simulink model "case9"  (R2024b)
settings: Solver=FixedStepAuto  StartTime=0  StopTime=1  FixedStep=1e-7  RelTol=1e-3
values from neighbouring files (symbols this model uses):
  SG_D_1_D = 0.01056    [IEEE9_case_parameters.m]    (also in case1_parameters.m; case2_parameters.m; case3_parameters.m; case4_parameters.m)
  SG_D_1_EnableSaturation = 0    [IEEE9_case_parameters.m]    (also in case1_parameters.m; case2_parameters.m; case3_parameters.m; case4_parameters.m)
  SG_D_1_f0 = 60    [IEEE9_case_parameters.m]    (also in case1_parameters.m; case2_parameters.m; case3_parameters.m; case4_parameters.m)
  SG_D_1_H = 7.5    [IEEE9_case_parameters.m]    (also in case1_parameters.m; case2_parameters.m; case3_parameters.m; case4_parameters.m)
  SG_D_1_K_A = 20    [IEEE9_case_parameters.m]    (also in case1_parameters.m; case2_parameters.m; case3_parameters.m; case4_parameters.m)
  SG_D_1_K_E = 1.000000e+1    (= 10)    [IEEE9_case_parameters.m]    (also in case1_parameters.m; case2_parameters.m; case3_parameters.m; case4_parameters.m)
  SG_D_1_K_F = 2.363    [IEEE9_case_parameters.m]    (also in case1_parameters.m; case2_parameters.m; case3_parameters.m; case4_parameters.m)
  SG_D_1_K_s = 0.5    [IEEE9_case_parameters.m]    (also in case1_parameters.m = 5; case2_parameters.m = 5; case3_parameters.m = 5; case4_parameters.m = 5)
  SG_D_1_R_a = 0.001088    [IEEE9_case_parameters.m]    (also in case1_parameters.m; case2_parameters.m; case3_parameters.m; case4_parameters.m)
  SG_D_1_S_A = 1    [IEEE9_case_parameters.m]    (also in case1_parameters.m; case2_parameters.m; case3_parameters.m; case4_parameters.m)
  SG_D_1_S_B = 0.103    [IEEE9_case_parameters.m]    (also in case1_parameters.m; case2_parameters.m; case3_parameters.m; case4_parameters.m)
  SG_D_1_S_N = 10.659857    [IEEE9_case_parameters.m]    (also in case1_parameters.m; case2_parameters.m; case3_parameters.m; case4_parameters.m)
  SG_D_1_SpeedPara = 200    [IEEE9_case_parameters.m]    (also in case1_parameters.m; case2_parameters.m; case3_parameters.m; case4_parameters.m)
  SG_D_1_T_0 = 0.720173    [IEEE9_case_parameters.m]    (also in case1_parameters.m = 0.755522; case2_parameters.m = 0.808931; case3_parameters.m = 0.869402; case4_parameters.m = 0.729316)
  SG_D_1_T_1 = 0.3    [IEEE9_case_parameters.m]    (also in case1_parameters.m; case2_parameters.m; case3_parameters.m; case4_parameters.m)
  SG_D_1_T_2 = 0.05    [IEEE9_case_parameters.m]    (also in case1_parameters.m; case2_parameters.m; case3_parameters.m; case4_parameters.m)
  SG_D_1_T_3 = 0.02    [IEEE9_case_parameters.m]    (also in case1_parameters.m; case2_parameters.m; case3_parameters.m; case4_parameters.m)
  SG_D_1_T_4 = 0.005    [IEEE9_case_parameters.m]    (also in case1_parameters.m; case2_parameters.m; case3_parameters.m; case4_parameters.m)
  SG_D_1_T_A = 0.02    [IEEE9_case_parameters.m]    (also in case1_parameters.m; case2_parameters.m; case3_parameters.m; case4_parameters.m)
  SG_D_1_T_dd = 8.000000e+0    (= 8)    [IEEE9_case_parameters.m]    (also in case1_parameters.m; case2_parameters.m; case3_parameters.m; case4_parameters.m)
  SG_D_1_T_ddd = 0.04    [IEEE9_case_parameters.m]    (also in case1_parameters.m; case2_parameters.m; case3_parameters.m; case4_parameters.m)
  SG_D_1_T_E = 0.314    [IEEE9_case_parameters.m]    (also in case1_parameters.m; case2_parameters.m; case3_parameters.m; case4_parameters.m)
  SG_D_1_T_F = 0.35    [IEEE9_case_parameters.m]    (also in case1_parameters.m; case2_parameters.m; case3_parameters.m; case4_parameters.m)
  SG_D_1_T_qd = 0.8    [IEEE9_case_parameters.m]    (also in case1_parameters.m; case2_parameters.m; case3_parameters.m; case4_parameters.m)
  SG_D_1_T_qdd = 0.02    [IEEE9_case_parameters.m]    (also in case1_parameters.m; case2_parameters.m; case3_parameters.m; case4_parameters.m)
  SG_D_1_T_speed = 0.1    [IEEE9_case_parameters.m]    (also in case1_parameters.m = 200; case2_parameters.m = 200; case3_parameters.m = 200; case4_parameters.m = 200)
  SG_D_1_T_w = 0.5    [IEEE9_case_parameters.m]    (also in case1_parameters.m; case2_parameters.m; case3_parameters.m; case4_parameters.m)
  SG_D_1_V_ref = 1.990276    [IEEE9_case_parameters.m]    (also in case1_parameters.m = 2.042296; case2_parameters.m = 2.051388; case3_parameters.m = 2.089584; case4_parameters.m = 2.01845)
  SG_D_1_w_ref = 376.991118    [IEEE9_case_parameters.m]    (also in case1_parameters.m; case2_parameters.m; case3_parameters.m; case4_parameters.m)
  SG_D_1_wb = 6.000000e+1    (= 60)    [IEEE9_case_parameters.m]    (also in case1_parameters.m; case2_parameters.m; case3_parameters.m; case4_parameters.m)
  SG_D_1_x_d = 1.9    [IEEE9_case_parameters.m]    (also in case1_parameters.m; case2_parameters.m; case3_parameters.m; case4_parameters.m)
  SG_D_1_x_dd = 0.302    [IEEE9_case_parameters.m]    (also in case1_parameters.m; case2_parameters.m; case3_parameters.m; case4_parameters.m)
  SG_D_1_x_ddd = 0.204    [IEEE9_case_parameters.m]    (also in case1_parameters.m; case2_parameters.m; case3_parameters.m; case4_parameters.m)
  SG_D_1_x_l = 0.05    [IEEE9_case_parameters.m]    (also in case1_parameters.m; case2_parameters.m; case3_parameters.m; case4_parameters.m)
  SG_D_1_x_q = 1.3    [IEEE9_case_parameters.m]    (also in case1_parameters.m; case2_parameters.m; case3_parameters.m; case4_parameters.m)
  SG_D_1_x_qd = 0.5    [IEEE9_case_parameters.m]    (also in case1_parameters.m; case2_parameters.m; case3_parameters.m; case4_parameters.m)
  SG_D_1_x_qdd = 0.3    [IEEE9_case_parameters.m]    (also in case1_parameters.m; case2_parameters.m; case3_parameters.m; case4_parameters.m)
  SG_D_2_D = 0.02    [IEEE9_case_parameters.m]    (also in case1_parameters.m; case2_parameters.m; case3_parameters.m; case4_parameters.m)
  SG_D_2_EnableSaturation = 0    [IEEE9_case_parameters.m]    (also in case1_parameters.m; case2_parameters.m; case3_parameters.m; case4_parameters.m)
  SG_D_2_f0 = 60    [IEEE9_case_parameters.m]    (also in case1_parameters.m; case2_parameters.m; case3_parameters.m; case4_parameters.m)
  SG_D_2_H = 8.000000e+0    (= 8)    [IEEE9_case_parameters.m]    (also in case1_parameters.m; case2_parameters.m; case3_parameters.m; case4_parameters.m)
  SG_D_2_K_A = 20    [IEEE9_case_parameters.m]    (also in case1_parameters.m; case2_parameters.m; case3_parameters.m; case4_parameters.m)
  SG_D_2_K_E = 1.000000e+1    (= 10)    [IEEE9_case_parameters.m]    (also in case1_parameters.m; case2_parameters.m; case3_parameters.m; case4_parameters.m)
  SG_D_2_K_F = 2.363    [IEEE9_case_parameters.m]    (also in case1_parameters.m; case2_parameters.m; case3_parameters.m; case4_parameters.m)
  SG_D_2_K_s = 0.5    [IEEE9_case_parameters.m]    (also in case1_parameters.m = 4; case2_parameters.m = 4; case3_parameters.m = 4; case4_parameters.m = 4)
  SG_D_2_R_a = 0.001088    [IEEE9_case_parameters.m]    (also in case1_parameters.m; case2_parameters.m; case3_parameters.m; case4_parameters.m)
  SG_D_2_S_A = 1    [IEEE9_case_parameters.m]    (also in case1_parameters.m; case2_parameters.m; case3_parameters.m; case4_parameters.m)
  SG_D_2_S_B = 0.103    [IEEE9_case_parameters.m]    (also in case1_parameters.m; case2_parameters.m; case3_parameters.m; case4_parameters.m)
  SG_D_2_S_N = 10.659857    [IEEE9_case_parameters.m]    (also in case1_parameters.m; case2_parameters.m; case3_parameters.m; case4_parameters.m)
  SG_D_2_SpeedPara = 200    [IEEE9_case_parameters.m]    (also in case1_parameters.m; case2_parameters.m; case3_parameters.m; case4_parameters.m)
  SG_D_2_T_0 = 1.632913    [IEEE9_case_parameters.m]    (also in case1_parameters.m = 1.632925; case2_parameters.m = 1.632915; case3_parameters.m = 1.632914; case4_parameters.m = 1.632927)
  SG_D_2_T_1 = 0.2    [IEEE9_case_parameters.m]    (also in case1_parameters.m; case2_parameters.m; case3_parameters.m; case4_parameters.m)
  SG_D_2_T_2 = 0.05    [IEEE9_case_parameters.m]    (also in case1_parameters.m; case2_parameters.m; case3_parameters.m; case4_parameters.m)
  SG_D_2_T_3 = 0.02    [IEEE9_case_parameters.m]    (also in case1_parameters.m; case2_parameters.m; case3_parameters.m; case4_parameters.m)
  SG_D_2_T_4 = 0.005    [IEEE9_case_parameters.m]    (also in case1_parameters.m; case2_parameters.m; case3_parameters.m; case4_parameters.m)
  SG_D_2_T_A = 0.02    [IEEE9_case_parameters.m]    (also in case1_parameters.m; case2_parameters.m; case3_parameters.m; case4_parameters.m)
  SG_D_2_T_dd = 7.9    [IEEE9_case_parameters.m]    (also in case1_parameters.m; case2_parameters.m; case3_parameters.m; case4_parameters.m)
  SG_D_2_T_ddd = 0.04    [IEEE9_case_parameters.m]    (also in case1_parameters.m; case2_parameters.m; case3_parameters.m; case4_parameters.m)
  SG_D_2_T_E = 0.314    [IEEE9_case_parameters.m]    (also in case1_parameters.m; case2_parameters.m; case3_parameters.m; case4_parameters.m)
  SG_D_2_T_F = 0.35    [IEEE9_case_parameters.m]    (also in case1_parameters.m; case2_parameters.m; case3_parameters.m; case4_parameters.m)
  SG_D_2_T_qd = 0.8    [IEEE9_case_parameters.m]    (also in case1_parameters.m; case2_parameters.m; case3_parameters.m; case4_parameters.m)
  SG_D_2_T_qdd = 0.015    [IEEE9_case_parameters.m]    (also in case1_parameters.m; case2_parameters.m; case3_parameters.m; case4_parameters.m)
  SG_D_2_T_speed = 0.1    [IEEE9_case_parameters.m]    (also in case1_parameters.m = 150; case2_parameters.m = 150; case3_parameters.m = 150; case4_parameters.m = 150)
  SG_D_2_T_w = 0.35    [IEEE9_case_parameters.m]    (also in case1_parameters.m; case2_parameters.m; case3_parameters.m; case4_parameters.m)
  SG_D_2_V_ref = 2.58547    [IEEE9_case_parameters.m]    (also in case1_parameters.m = 2.597896; case2_parameters.m = 2.587136; case3_parameters.m = 2.586042; case4_parameters.m = 2.599679)
  SG_D_2_w_ref = 376.991118    [IEEE9_case_parameters.m]    (also in case1_parameters.m; case2_parameters.m; case3_parameters.m; case4_parameters.m)
  SG_D_2_wb = 6.000000e+1    (= 60)    [IEEE9_case_parameters.m]    (also in case1_parameters.m; case2_parameters.m; case3_parameters.m; case4_parameters.m)
  SG_D_2_x_d = 1.8    [IEEE9_case_parameters.m]    (also in case1_parameters.m; case2_parameters.m; case3_parameters.m; case4_parameters.m)
  SG_D_2_x_dd = 0.302    [IEEE9_case_parameters.m]    (also in case1_parameters.m; case2_parameters.m; case3_parameters.m; case4_parameters.m)
  SG_D_2_x_ddd = 0.204    [IEEE9_case_parameters.m]    (also in case1_parameters.m; case2_parameters.m; case3_parameters.m; case4_parameters.m)
  SG_D_2_x_l = 0.05    [IEEE9_case_parameters.m]    (also in case1_parameters.m; case2_parameters.m; case3_parameters.m; case4_parameters.m)
  SG_D_2_x_q = 1.25    [IEEE9_case_parameters.m]    (also in case1_parameters.m; case2_parameters.m; case3_parameters.m; case4_parameters.m)
  SG_D_2_x_qd = 0.5    [IEEE9_case_parameters.m]    (also in case1_parameters.m; case2_parameters.m; case3_parameters.m; case4_parameters.m)
  SG_D_2_x_qdd = 0.3    [IEEE9_case_parameters.m]    (also in case1_parameters.m; case2_parameters.m; case3_parameters.m; case4_parameters.m)
  SG_D_3_D = 0.02    [IEEE9_case_parameters.m]    (also in case1_parameters.m; case2_parameters.m; case3_parameters.m; case4_parameters.m)
  SG_D_3_EnableSaturation = 0    [IEEE9_case_parameters.m]    (also in case1_parameters.m; case2_parameters.m; case3_parameters.m; case4_parameters.m)
  SG_D_3_f0 = 60    [IEEE9_case_parameters.m]    (also in case1_parameters.m; case2_parameters.m; case3_parameters.m; case4_parameters.m)
  SG_D_3_H = 7.7    [IEEE9_case_parameters.m]    (also in case1_parameters.m; case2_parameters.m; case3_parameters.m; case4_parameters.m)
  SG_D_3_K_A = 20    [IEEE9_case_parameters.m]    (also in case1_parameters.m; case2_parameters.m; case3_parameters.m; case4_parameters.m)
  SG_D_3_K_E = 1.000000e+1    (= 10)    [IEEE9_case_parameters.m]    (also in case1_parameters.m; case2_parameters.m; case3_parameters.m; case4_parameters.m)
  SG_D_3_K_F = 2.363    [IEEE9_case_parameters.m]    (also in case1_parameters.m; case2_parameters.m; case3_parameters.m; case4_parameters.m)
  SG_D_3_K_s = 0.2    [IEEE9_case_parameters.m]    (also in case1_parameters.m = 2; case2_parameters.m = 2; case3_parameters.m = 2; case4_parameters.m = 2)
  SG_D_3_R_a = 0.001088    [IEEE9_case_parameters.m]    (also in case1_parameters.m; case2_parameters.m; case3_parameters.m; case4_parameters.m)
  SG_D_3_S_A = 1    [IEEE9_case_parameters.m]    (also in case1_parameters.m; case2_parameters.m; case3_parameters.m; case4_parameters.m)
  SG_D_3_S_B = 0.103    [IEEE9_case_parameters.m]    (also in case1_parameters.m; case2_parameters.m; case3_parameters.m; case4_parameters.m)
  SG_D_3_S_N = 10.659857    [IEEE9_case_parameters.m]    (also in case1_parameters.m; case2_parameters.m; case3_parameters.m; case4_parameters.m)
  SG_D_3_SpeedPara = 200    [IEEE9_case_parameters.m]    (also in case1_parameters.m; case2_parameters.m; case3_parameters.m; case4_parameters.m)
  SG_D_3_T_0 = 0.850788    [IEEE9_case_parameters.m]    (also in case1_parameters.m = 0.850786; case2_parameters.m = 0.850787; case3_parameters.m; case4_parameters.m = 0.850786)
  SG_D_3_T_1 = 0.2    [IEEE9_case_parameters.m]    (also in case1_parameters.m; case2_parameters.m; case3_parameters.m; case4_parameters.m)
  SG_D_3_T_2 = 0.05    [IEEE9_case_parameters.m]    (also in case1_parameters.m; case2_parameters.m; case3_parameters.m; case4_parameters.m)
  SG_D_3_T_3 = 0.02    [IEEE9_case_parameters.m]    (also in case1_parameters.m; case2_parameters.m; case3_parameters.m; case4_parameters.m)
  SG_D_3_T_4 = 0.005    [IEEE9_case_parameters.m]    (also in case1_parameters.m; case2_parameters.m; case3_parameters.m; case4_parameters.m)
  SG_D_3_T_A = 0.02    [IEEE9_case_parameters.m]    (also in case1_parameters.m; case2_parameters.m; case3_parameters.m; case4_parameters.m)
  SG_D_3_T_dd = 8.1    [IEEE9_case_parameters.m]    (also in case1_parameters.m; case2_parameters.m; case3_parameters.m; case4_parameters.m)
  SG_D_3_T_ddd = 0.04    [IEEE9_case_parameters.m]    (also in case1_parameters.m; case2_parameters.m; case3_parameters.m; case4_parameters.m)
  SG_D_3_T_E = 0.314    [IEEE9_case_parameters.m]    (also in case1_parameters.m; case2_parameters.m; case3_parameters.m; case4_parameters.m)
  SG_D_3_T_F = 0.35    [IEEE9_case_parameters.m]    (also in case1_parameters.m; case2_parameters.m; case3_parameters.m; case4_parameters.m)
  SG_D_3_T_qd = 0.8    [IEEE9_case_parameters.m]    (also in case1_parameters.m; case2_parameters.m; case3_parameters.m; case4_parameters.m)
  SG_D_3_T_qdd = 0.015    [IEEE9_case_parameters.m]    (also in case1_parameters.m; case2_parameters.m; case3_parameters.m; case4_parameters.m)
  SG_D_3_T_speed = 0.1    [IEEE9_case_parameters.m]    (also in case1_parameters.m = 180; case2_parameters.m = 180; case3_parameters.m = 180; case4_parameters.m = 180)
  SG_D_3_T_w = 0.4    [IEEE9_case_parameters.m]    (also in case1_parameters.m; case2_parameters.m; case3_parameters.m; case4_parameters.m)
  SG_D_3_V_ref = 1.892727    [IEEE9_case_parameters.m]    (also in case1_parameters.m = 1.906439; case2_parameters.m = 1.895535; case3_parameters.m = 1.892105; case4_parameters.m = 1.906598)
  SG_D_3_w_ref = 376.991118    [IEEE9_case_parameters.m]    (also in case1_parameters.m; case2_parameters.m; case3_parameters.m; case4_parameters.m)
  SG_D_3_wb = 6.000000e+1    (= 60)    [IEEE9_case_parameters.m]    (also in case1_parameters.m; case2_parameters.m; case3_parameters.m; case4_parameters.m)
  SG_D_3_x_d = 1.85    [IEEE9_case_parameters.m]    (also in case1_parameters.m; case2_parameters.m; case3_parameters.m; case4_parameters.m)
  SG_D_3_x_dd = 0.302    [IEEE9_case_parameters.m]    (also in case1_parameters.m; case2_parameters.m; case3_parameters.m; case4_parameters.m)
  SG_D_3_x_ddd = 0.204    [IEEE9_case_parameters.m]    (also in case1_parameters.m; case2_parameters.m; case3_parameters.m; case4_parameters.m)
  SG_D_3_x_l = 0.05    [IEEE9_case_parameters.m]    (also in case1_parameters.m; case2_parameters.m; case3_parameters.m; case4_parameters.m)
  SG_D_3_x_q = 1.2    [IEEE9_case_parameters.m]    (also in case1_parameters.m; case2_parameters.m; case3_parameters.m; case4_parameters.m)
  SG_D_3_x_qd = 0.5    [IEEE9_case_parameters.m]    (also in case1_parameters.m; case2_parameters.m; case3_parameters.m; case4_parameters.m)
  SG_D_3_x_qdd = 0.3    [IEEE9_case_parameters.m]    (also in case1_parameters.m; case2_parameters.m; case3_parameters.m; case4_parameters.m)
(part 6 of 12)

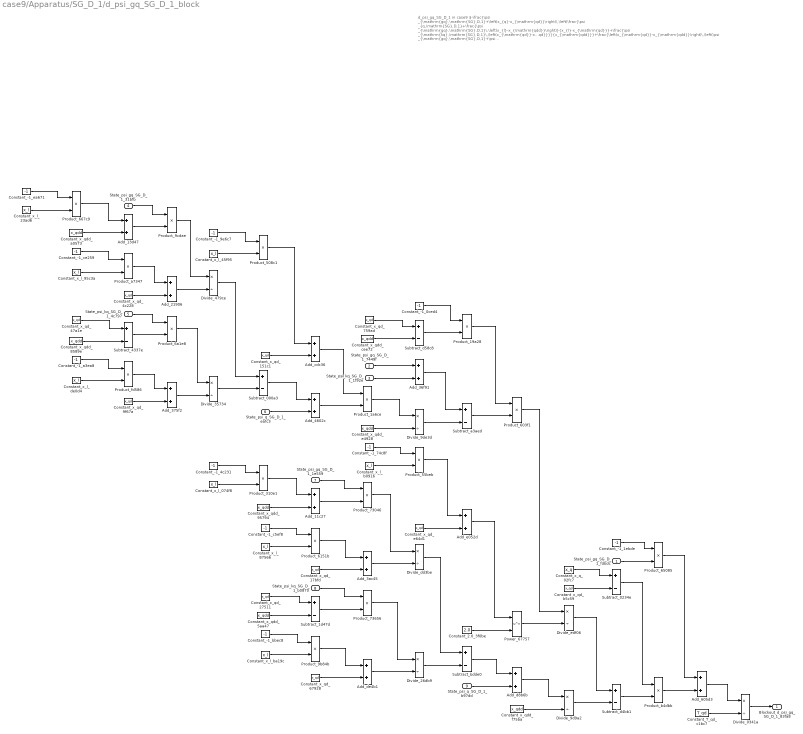
== system case9/Apparatus/SG_D_1/d_psi_gq_SG_D_1_block ==
  note: d_psi_gq_SG_D_1 in case9
      | $-\frac{\psi _{\mathrm{gq},\mathrm{SG},D,1}+\left(x_{q}-x_{\mathrm{qd}}\right)\,\left(\frac{\psi _{q,\mathrm{SG},D,1}+\frac{\psi _{\mathrm{gq},\mathrm{SG},D,1}\,\left(x_{l}-x_{\mathrm{qdd}}\right)}{x_{l}-x_{\mathrm{qd}}}+\frac{\psi _{\mathrm{kq},\mathrm{SG},D,1}\,\left(x_{\mathrm{qd}}-x_{\mathrm{qdd}}\right)}{x_{l}-x_{\mathrm{qd}}}}{x_{\mathrm{qdd}}}+\frac{\left(x_{\mathrm{qd}}-x_{\mathrm{qdd}}\right)\,\left(\psi _{\mathrm{gq},\mathrm{SG},D,1}+\psi _{\mathrm{kq},\mathrm{SG},D,1}+\frac{\left(x_{l}-x_{\mathrm{qd}}\right)\,\left(\psi _{q,\mathrm{SG},D,1}+\frac{\psi _{\mathrm{gq},\mathrm{SG},D,1}\,\left(x_{l}-x_{\mathrm{qdd}}\right)}{x_{l}-x_{\mathrm{qd}}}+\frac{\psi _{\mathrm{kq},\mathrm{SG},D,1}\,\left(x_{\mathrm{qd}}-x_{\mathrm{qdd}}\right)}{x_{l}-x_{\mathrm{qd}}}\right)}{x_{\mathrm{qdd}}}\right)}{{\left(x_{l}-x_{\mathrm{qd}}\right)}^2}\right)}{T_{\mathrm{qd}}}$
      | Automatically generated on 2025-10-31 19:34:40 .
  State_psi_gq_SG_D_1_fdbdc : Inport
  State_psi_gq_SG_D_1_7449f : Inport  Port=2
  State_psi_kq_SG_D_1_1f92e : Inport  Port=3
  State_psi_gq_SG_D_1_31bfb : Inport  Port=4
  State_psi_kq_SG_D_1_4c797 : Inport  Port=5
  State_psi_q_SG_D_1_eafc3 : Inport  Port=6
  State_psi_gq_SG_D_1_1e559 : Inport  Port=7
  State_psi_kq_SG_D_1_b0870 : Inport  Port=8
  State_psi_q_SG_D_1_b97dd : Inport  Port=9
  Add_11c27 : Sum
  Add_13d47 : Sum
  Add_21906 : Sum
  Add_36f91 : Sum
  Add_375f2 : Sum
  Add_3ac45 : Sum
  Add_4602c : Sum
  Add_605d3 : Sum
  Add_cdc36 : Sum
  Add_d8b6b : Sum
  Add_de4b1 : Sum
  Add_e052d : Sum
  Constant_-1_0ced4 : Constant  Value=-1
  Constant_-1_1ebde : Constant  Value=-1
  Constant_-1_4c231 : Constant  Value=-1
  Constant_-1_74c8f : Constant  Value=-1
  Constant_-1_9e6c7 : Constant  Value=-1
  Constant_-1_a3ea8 : Constant  Value=-1
  Constant_-1_bbec8 : Constant  Value=-1
  Constant_-1_c5ef8 : Constant  Value=-1
  Constant_-1_ce259 : Constant  Value=-1
  Constant_-1_ea671 : Constant  Value=-1
  Constant_2.0_3f0be : Constant  Value=2.0
  Constant_T_qd_c1bc7 : Constant  Value=T_qd
  Constant_x_l_074f8 : Constant  Value=x_l
  Constant_x_l_23ad6 : Constant  Value=x_l
  Constant_x_l_45f95 : Constant  Value=x_l
  Constant_x_l_87566 : Constant  Value=x_l
  Constant_x_l_95c3a : Constant  Value=x_l
  Constant_x_l_b0916 : Constant  Value=x_l
  Constant_x_l_ba19c : Constant  Value=x_l
  Constant_x_l_de0d4 : Constant  Value=x_l
  Constant_x_q_02fc7 : Constant  Value=x_q
  Constant_x_qd_151c1 : Constant  Value=x_qd
  Constant_x_qd_17bfd : Constant  Value=x_qd
  Constant_x_qd_27511 : Constant  Value=x_qd
  Constant_x_qd_47a1e : Constant  Value=x_qd
  Constant_x_qd_4c228 : Constant  Value=x_qd
  Constant_x_qd_67928 : Constant  Value=x_qd
  Constant_x_qd_759ad : Constant  Value=x_qd
  Constant_x_qd_9f67a : Constant  Value=x_qd
  Constant_x_qd_b5c59 : Constant  Value=x_qd
  Constant_x_qd_e64d1 : Constant  Value=x_qd
  Constant_x_qdd_5aa47 : Constant  Value=x_qdd
  Constant_x_qdd_8589e : Constant  Value=x_qdd
  Constant_x_qdd_95794 : Constant  Value=x_qdd
  Constant_x_qdd_a0573 : Constant  Value=x_qdd
  Constant_x_qdd_cee72 : Constant  Value=x_qdd
  Constant_x_qdd_e4928 : Constant  Value=x_qdd
  Constant_x_qdd_f75ba : Constant  Value=x_qdd
  Divide_0341a : Product  Inputs=*/
  Divide_26db9 : Product  Inputs=*/
  Divide_35734 : Product  Inputs=*/
  Divide_479ce : Product  Inputs=*/
  Divide_9d9a2 : Product  Inputs=*/
  Divide_9de3d : Product  Inputs=*/
  Divide_dd3be : Product  Inputs=*/
  Divide_edf06 : Product  Inputs=*/
  Power_67757 : Math  Operator=pow
  Product_19a28 : Product
  Product_1a6ce : Product
  Product_310e1 : Product
  Product_508c1 : Product
  Product_55beb : Product
  Product_603f1 : Product
  Product_6151b : Product
  Product_65085 : Product
  Product_667c9 : Product
  Product_6a1e8 : Product
  Product_73046 : Product
  Product_73656 : Product
  Product_9b84b : Product
  Product_9cdae : Product
  Product_a7347 : Product
  Product_b4dbb : Product
  Product_fd586 : Product
  Subtract_000a3 : Sum  Inputs=+-
  Subtract_0234e : Sum  Inputs=+-
  Subtract_1d47d : Sum  Inputs=+-
  Subtract_4337e : Sum  Inputs=+-
  Subtract_a3aed : Sum  Inputs=+-
  Subtract_bdde0 : Sum  Inputs=+-
  Subtract_d4bb1 : Sum  Inputs=+-
  Subtract_d58c8 : Sum  Inputs=+-
  Blockout_d_psi_gq_SG_D_1_83fa8 : Outport
  wires:
  State_psi_gq_SG_D_1_31bfb/1 -> Product_9cdae/1
  Constant_-1_ce259/1 -> Product_a7347/1
  Divide_479ce/1 -> Subtract_000a3/1
  Add_21906/1 -> Divide_479ce/2
  Product_667c9/1 -> Add_13d47/1
  Constant_x_qd_151c1/1 -> Add_cdc36/2
  Constant_-1_ea671/1 -> Product_667c9/1
  Constant_x_qdd_a0573/1 -> Add_13d47/2
  Constant_x_l_95c3a/1 -> Product_a7347/2
  Constant_x_l_23ad6/1 -> Product_667c9/2
  Constant_-1_a3ea8/1 -> Product_fd586/1
  Constant_x_qd_47a1e/1 -> Subtract_4337e/1
  Constant_x_qdd_e4928/1 -> Divide_9de3d/2
  Constant_x_l_de0d4/1 -> Product_fd586/2
  Constant_x_qdd_8589e/1 -> Subtract_4337e/2
  Subtract_000a3/1 -> Add_4602c/1
  Add_13d47/1 -> Product_9cdae/2
  Product_9cdae/1 -> Divide_479ce/1
  Product_a7347/1 -> Add_21906/1
  Constant_x_qd_4c228/1 -> Add_21906/2
  State_psi_kq_SG_D_1_4c797/1 -> Product_6a1e8/1
  Product_fd586/1 -> Add_375f2/1
  Subtract_4337e/1 -> Product_6a1e8/2
  Constant_x_qd_9f67a/1 -> Add_375f2/2
  Product_6a1e8/1 -> Divide_35734/1
  Add_375f2/1 -> Divide_35734/2
  Constant_-1_0ced4/1 -> Product_19a28/1
  Constant_-1_9e6c7/1 -> Product_508c1/1
  Add_3ac45/1 -> Divide_dd3be/2
  Product_9b84b/1 -> Add_de4b1/1
  Subtract_1d47d/1 -> Product_73656/2
  Constant_x_l_45f95/1 -> Product_508c1/2
  Divide_35734/1 -> Subtract_000a3/2
  Subtract_0234e/1 -> Product_b4dbb/1
  Constant_-1_74c8f/1 -> Product_55beb/1
  Constant_-1_4c231/1 -> Product_310e1/1
  Constant_x_l_b0916/1 -> Product_55beb/2
  Constant_x_l_074f8/1 -> Product_310e1/2
  Constant_x_qd_17bfd/1 -> Add_3ac45/2
  Product_508c1/1 -> Add_cdc36/1
  State_psi_q_SG_D_1_eafc3/1 -> Add_4602c/2
  Product_310e1/1 -> Add_11c27/1
  Constant_x_qdd_95794/1 -> Add_11c27/2
  Constant_-1_c5ef8/1 -> Product_6151b/1
  Constant_x_qd_67928/1 -> Add_de4b1/2
  Add_cdc36/1 -> Product_1a6ce/1
  Constant_x_l_87566/1 -> Product_6151b/2
  Constant_-1_bbec8/1 -> Product_9b84b/1
  Constant_x_qd_27511/1 -> Subtract_1d47d/1
  Product_1a6ce/1 -> Divide_9de3d/1
  Constant_x_l_ba19c/1 -> Product_9b84b/2
  Divide_edf06/1 -> Subtract_d4bb1/1
  Constant_x_qdd_5aa47/1 -> Subtract_1d47d/2
  Add_4602c/1 -> Product_1a6ce/2
  State_psi_gq_SG_D_1_1e559/1 -> Product_73046/1
  Add_11c27/1 -> Product_73046/2
  Product_6151b/1 -> Add_3ac45/1
  State_psi_kq_SG_D_1_b0870/1 -> Product_73656/1
  Add_de4b1/1 -> Divide_26db9/2
  State_psi_gq_SG_D_1_7449f/1 -> Add_36f91/1
  Constant_x_qd_759ad/1 -> Subtract_d58c8/1
  Constant_x_qdd_cee72/1 -> Subtract_d58c8/2
  Product_73656/1 -> Divide_26db9/1
  State_psi_kq_SG_D_1_1f92e/1 -> Add_36f91/2
  Product_73046/1 -> Divide_dd3be/1
  Subtract_d58c8/1 -> Product_19a28/2
  Add_36f91/1 -> Subtract_a3aed/1
  Divide_9de3d/1 -> Subtract_a3aed/2
  Product_55beb/1 -> Add_e052d/1
  Constant_x_qd_e64d1/1 -> Add_e052d/2
  Divide_dd3be/1 -> Subtract_bdde0/1
  Divide_26db9/1 -> Subtract_bdde0/2
  Product_19a28/1 -> Product_603f1/1
  Subtract_a3aed/1 -> Product_603f1/2
  Add_e052d/1 -> Power_67757/1
  Constant_2.0_3f0be/1 -> Power_67757/2
  Subtract_bdde0/1 -> Add_d8b6b/1
  State_psi_q_SG_D_1_b97dd/1 -> Add_d8b6b/2
  Product_603f1/1 -> Divide_edf06/1
  Power_67757/1 -> Divide_edf06/2
  Add_d8b6b/1 -> Divide_9d9a2/1
  Constant_x_qdd_f75ba/1 -> Divide_9d9a2/2
  Constant_x_q_02fc7/1 -> Subtract_0234e/1
  Constant_x_qd_b5c59/1 -> Subtract_0234e/2
  Divide_9d9a2/1 -> Subtract_d4bb1/2
  Constant_-1_1ebde/1 -> Product_65085/1
  State_psi_gq_SG_D_1_fdbdc/1 -> Product_65085/2
  Subtract_d4bb1/1 -> Product_b4dbb/2
  Product_65085/1 -> Add_605d3/1
  Product_b4dbb/1 -> Add_605d3/2
  Add_605d3/1 -> Divide_0341a/1
  Constant_T_qd_c1bc7/1 -> Divide_0341a/2
  Divide_0341a/1 -> Blockout_d_psi_gq_SG_D_1_83fa8/1

== system case9/Apparatus/SG_D_1/d_psi_kq_SG_D_1_block ==
  note: d_psi_kq_SG_D_1 in case9
      | $-\frac{\psi _{\mathrm{gq},\mathrm{SG},D,1}+\psi _{\mathrm{kq},\mathrm{SG},D,1}+\frac{\left(x_{l}-x_{\mathrm{qd}}\right)\,\left(\psi _{q,\mathrm{SG},D,1}+\frac{\psi _{\mathrm{gq},\mathrm{SG},D,1}\,\left(x_{l}-x_{\mathrm{qdd}}\right)}{x_{l}-x_{\mathrm{qd}}}+\frac{\psi _{\mathrm{kq},\mathrm{SG},D,1}\,\left(x_{\mathrm{qd}}-x_{\mathrm{qdd}}\right)}{x_{l}-x_{\mathrm{qd}}}\right)}{x_{\mathrm{qdd}}}}{T_{\mathrm{qdd}}}$
      | Automatically generated on 2025-10-31 19:34:41 .
  State_psi_gq_SG_D_1_20359 : Inport
  State_psi_kq_SG_D_1_02235 : Inport  Port=2
  State_psi_gq_SG_D_1_5b14b : Inport  Port=3
  State_psi_kq_SG_D_1_1396d : Inport  Port=4
  State_psi_q_SG_D_1_e7314 : Inport  Port=5
  Add_06458 : Sum
  Add_873c5 : Sum
  Add_945ca : Sum
  Add_95636 : Sum
  Add_a65ed : Sum
  Add_bc1c6 : Sum
  Constant_-1_4b348 : Constant  Value=-1
  Constant_-1_66d13 : Constant  Value=-1
  Constant_-1_7eae6 : Constant  Value=-1
  Constant_-1_b006a : Constant  Value=-1
  Constant_-1_fe53d : Constant  Value=-1
  Constant_T_qdd_5e4e9 : Constant  Value=T_qdd
  Constant_x_l_2eef6 : Constant  Value=x_l
  Constant_x_l_461f2 : Constant  Value=x_l
  Constant_x_l_559ed : Constant  Value=x_l
  Constant_x_l_a9a58 : Constant  Value=x_l
  Constant_x_qd_1a100 : Constant  Value=x_qd
  Constant_x_qd_67afc : Constant  Value=x_qd
  Constant_x_qd_edeff : Constant  Value=x_qd
  Constant_x_qd_fdf31 : Constant  Value=x_qd
  Constant_x_qdd_400b6 : Constant  Value=x_qdd
  Constant_x_qdd_692c4 : Constant  Value=x_qdd
  Constant_x_qdd_be4c0 : Constant  Value=x_qdd
  Divide_2b43f : Product  Inputs=*/
  Divide_71da8 : Product  Inputs=*/
  Divide_bf59b : Product  Inputs=*/
  Divide_f6de6 : Product  Inputs=*/
  Product_0ba77 : Product
  Product_17ebc : Product
  Product_25d03 : Product
  Product_4de9c : Product
  Product_5fbf3 : Product
  Product_913de : Product
  Product_c66f6 : Product
  Product_d3303 : Product
  Subtract_28a94 : Sum  Inputs=+-
  Subtract_7a2c0 : Sum  Inputs=+-
  Subtract_9b8fd : Sum  Inputs=+-
  Blockout_d_psi_kq_SG_D_1_1846f : Outport
  wires:
  Product_25d03/1 -> Add_95636/1
  Constant_-1_66d13/1 -> Product_25d03/1
  Constant_x_l_2eef6/1 -> Product_25d03/2
  Constant_x_qdd_400b6/1 -> Add_95636/2
  Constant_-1_4b348/1 -> Product_d3303/1
  Constant_x_qd_1a100/1 -> Subtract_28a94/1
  Constant_x_qd_fdf31/1 -> Add_945ca/2
  Constant_-1_b006a/1 -> Product_17ebc/1
  Constant_x_l_461f2/1 -> Product_d3303/2
  Constant_x_qdd_be4c0/1 -> Subtract_28a94/2
  Constant_x_qd_67afc/1 -> Add_bc1c6/2
  Constant_x_l_a9a58/1 -> Product_17ebc/2
  Subtract_9b8fd/1 -> Add_06458/1
  Product_5fbf3/1 -> Subtract_9b8fd/1
  State_psi_gq_SG_D_1_5b14b/1 -> Product_c66f6/1
  Add_95636/1 -> Product_c66f6/2
  Product_17ebc/1 -> Add_a65ed/1
  Constant_x_qd_edeff/1 -> Add_a65ed/2
  State_psi_kq_SG_D_1_1396d/1 -> Product_0ba77/1
  Product_d3303/1 -> Add_bc1c6/1
  Subtract_28a94/1 -> Product_0ba77/2
  Product_c66f6/1 -> Divide_f6de6/1
  Add_a65ed/1 -> Divide_f6de6/2
  Product_0ba77/1 -> Divide_71da8/1
  Add_bc1c6/1 -> Divide_71da8/2
  Constant_-1_7eae6/1 -> Product_4de9c/1
  Constant_x_l_559ed/1 -> Product_4de9c/2
  Divide_f6de6/1 -> Subtract_7a2c0/1
  Divide_71da8/1 -> Subtract_7a2c0/2
  Product_4de9c/1 -> Add_945ca/1
  Add_873c5/1 -> Product_913de/2
  Subtract_7a2c0/1 -> Add_873c5/1
  State_psi_q_SG_D_1_e7314/1 -> Add_873c5/2
  Constant_-1_fe53d/1 -> Product_5fbf3/1
  State_psi_gq_SG_D_1_20359/1 -> Product_5fbf3/2
  Divide_2b43f/1 -> Add_06458/2
  Product_913de/1 -> Divide_2b43f/1
  Add_945ca/1 -> Product_913de/1
  State_psi_kq_SG_D_1_02235/1 -> Subtract_9b8fd/2
  Constant_x_qdd_692c4/1 -> Divide_2b43f/2
  Add_06458/1 -> Divide_bf59b/1
  Constant_T_qdd_5e4e9/1 -> Divide_bf59b/2
  Divide_bf59b/1 -> Blockout_d_psi_kq_SG_D_1_1846f/1

== system case9/Apparatus/SG_D_1/d_psi_q_SG_D_1_block ==
  note: d_psi_q_SG_D_1 in case9
      | $2\,\pi \,f_{0}\,\left(v_{d,\mathrm{SG},D,1}\,\cos\left(\theta _{\mathrm{SG},D,1}\right)+v_{q,\mathrm{SG},D,1}\,\sin\left(\theta _{\mathrm{SG},D,1}\right)-\frac{R_{a}\,\left(\psi _{q,\mathrm{SG},D,1}+\frac{\psi _{\mathrm{gq},\mathrm{SG},D,1}\,\left(x_{l}-x_{\mathrm{qdd}}\right)}{x_{l}-x_{\mathrm{qd}}}+\frac{\psi _{\mathrm{kq},\mathrm{SG},D,1}\,\left(x_{\mathrm{qd}}-x_{\mathrm{qdd}}\right)}{x_{l}-x_{\mathrm{qd}}}\right)}{x_{\mathrm{qdd}}}-\frac{\psi _{d,\mathrm{SG},D,1}\,w_{\mathrm{SG},D,1}}{2\,f_{0}\,\pi }\right)$
      | Automatically generated on 2025-10-31 19:34:37 .
  State_psi_gq_SG_D_1_e06cf : Inport
  State_psi_kq_SG_D_1_d4ed3 : Inport  Port=2
  State_psi_q_SG_D_1_8f107 : Inport  Port=3
  Input_v_d_SG_D_1_e85f7 : Inport  Port=4
  State_theta_SG_D_1_b63a1 : Inport  Port=5
  Input_v_q_SG_D_1_46a58 : Inport  Port=6
  State_theta_SG_D_1_fcbfe : Inport  Port=7
  State_psi_d_SG_D_1_9ece2 : Inport  Port=8
  State_w_SG_D_1_a0845 : Inport  Port=9
  Add_323c6 : Sum
  Add_583ae : Sum
  Add_6779d : Sum
  Add_6acf7 : Sum
  Add_b46b4 : Sum
  Constant_-1_024fb : Constant  Value=-1
  Constant_-1_6bd05 : Constant  Value=-1
  Constant_-1_9f485 : Constant  Value=-1
  Constant_-2.0_28195 : Constant  Value=-2.0
  Constant_2.0_387e6 : Constant  Value=2.0
  Constant_R_a_e430c : Constant  Value=R_a
  Constant_f0_73c2d : Constant  Value=f0
  Constant_f0_e8bd1 : Constant  Value=f0
  Constant_pi_9a496 : Constant  Value=pi
  Constant_pi_a35a0 : Constant  Value=pi
  Constant_x_l_7e967 : Constant  Value=x_l
  Constant_x_l_c6c0d : Constant  Value=x_l
  Constant_x_l_efad4 : Constant  Value=x_l
  Constant_x_qd_155b8 : Constant  Value=x_qd
  Constant_x_qd_2e84c : Constant  Value=x_qd
  Constant_x_qd_f4c16 : Constant  Value=x_qd
  Constant_x_qdd_91f68 : Constant  Value=x_qdd
  Constant_x_qdd_b22e8 : Constant  Value=x_qdd
  Constant_x_qdd_d86ff : Constant  Value=x_qdd
  Divide_09ba4 : Product  Inputs=*/
  Divide_15066 : Product  Inputs=*/
  Divide_3baef : Product  Inputs=*/
  Divide_3e22e : Product  Inputs=*/
  MathFunc_cos_5ad6c : Trigonometry  Operator=cos
  MathFunc_sin_42c9e : Trigonometry
  Product_2401e : Product
  Product_29cb7 : Product
  Product_2ec6b : Product
  Product_31a30 : Product
  Product_46fe9 : Product
  Product_4fd8e : Product
  Product_50d90 : Product
  Product_5e278 : Product
  Product_76f09 : Product
  Product_87948 : Product
  Product_8bfc0 : Product
  Product_97d6d : Product
  Product_c3375 : Product
  Product_f5b25 : Product
  Subtract_2f3d6 : Sum  Inputs=+-
  Subtract_e6a18 : Sum  Inputs=+-
  Subtract_ea955 : Sum  Inputs=+-
  Subtract_f36d7 : Sum  Inputs=+-
  Blockout_d_psi_q_SG_D_1_00fdb : Outport
  wires:
  Divide_3baef/1 -> Subtract_f36d7/1
  Product_76f09/1 -> Add_583ae/1
  Constant_x_l_c6c0d/1 -> Product_76f09/2
  Constant_-1_024fb/1 -> Product_76f09/1
  Constant_x_qdd_b22e8/1 -> Add_583ae/2
  Constant_x_l_7e967/1 -> Product_f5b25/2
  Constant_-1_9f485/1 -> Product_f5b25/1
  Constant_x_l_efad4/1 -> Product_97d6d/2
  Constant_x_qdd_91f68/1 -> Subtract_ea955/2
  State_psi_kq_SG_D_1_d4ed3/1 -> Product_8bfc0/1
  Constant_-1_6bd05/1 -> Product_97d6d/1
  Constant_x_qd_f4c16/1 -> Subtract_ea955/1
  State_psi_gq_SG_D_1_e06cf/1 -> Product_5e278/1
  Product_31a30/1 -> Blockout_d_psi_q_SG_D_1_00fdb/1
  Subtract_f36d7/1 -> Add_6acf7/1
  Product_5e278/1 -> Divide_3baef/1
  Add_583ae/1 -> Product_5e278/2
  Divide_3e22e/1 -> Subtract_f36d7/2
  Product_f5b25/1 -> Add_6779d/1
  Constant_x_qd_155b8/1 -> Add_6779d/2
  Constant_-2.0_28195/1 -> Product_c3375/1
  Product_8bfc0/1 -> Divide_3e22e/1
  Product_97d6d/1 -> Add_323c6/1
  Subtract_ea955/1 -> Product_8bfc0/2
  Constant_x_qd_2e84c/1 -> Add_323c6/2
  Add_6779d/1 -> Divide_3baef/2
  Add_323c6/1 -> Divide_3e22e/2
  Constant_f0_73c2d/1 -> Product_29cb7/2
  State_psi_q_SG_D_1_8f107/1 -> Add_6acf7/2
  Product_46fe9/1 -> Product_4fd8e/1
  Constant_R_a_e430c/1 -> Product_87948/1
  Product_4fd8e/1 -> Divide_09ba4/2
  Product_87948/1 -> Divide_15066/1
  Add_6acf7/1 -> Product_87948/2
  State_theta_SG_D_1_b63a1/1 -> MathFunc_cos_5ad6c/1
  Input_v_d_SG_D_1_e85f7/1 -> Product_2ec6b/1
  Constant_x_qdd_d86ff/1 -> Divide_15066/2
  MathFunc_cos_5ad6c/1 -> Product_2ec6b/2
  State_theta_SG_D_1_fcbfe/1 -> MathFunc_sin_42c9e/1
  Divide_15066/1 -> Subtract_2f3d6/1
  Constant_2.0_387e6/1 -> Product_46fe9/1
  State_w_SG_D_1_a0845/1 -> Product_2401e/2
  Constant_pi_9a496/1 -> Product_46fe9/2
  Subtract_e6a18/1 -> Add_b46b4/1
  Product_2ec6b/1 -> Subtract_2f3d6/2
  Divide_09ba4/1 -> Add_b46b4/2
  Input_v_q_SG_D_1_46a58/1 -> Product_50d90/1
  MathFunc_sin_42c9e/1 -> Product_50d90/2
  Product_50d90/1 -> Subtract_e6a18/2
  State_psi_d_SG_D_1_9ece2/1 -> Product_2401e/1
  Constant_f0_e8bd1/1 -> Product_4fd8e/2
  Constant_pi_a35a0/1 -> Product_c3375/2
  Subtract_2f3d6/1 -> Subtract_e6a18/1
  Product_2401e/1 -> Divide_09ba4/1
  Product_c3375/1 -> Product_29cb7/1
  Product_29cb7/1 -> Product_31a30/1
  Add_b46b4/1 -> Product_31a30/2

== system case9/Apparatus/SG_D_1/d_theta_SG_D_1_block ==
  note: d_theta_SG_D_1 in case9
      | $w_{\mathrm{SG},D,1}-2\,\pi \,f_{0}$
      | Automatically generated on 2025-10-31 19:34:43 .
  State_w_SG_D_1_c5d1e : Inport
  Add_b1f62 : Sum
  Constant_-2.0_b7139 : Constant  Value=-2.0
  Constant_f0_a2466 : Constant  Value=f0
  Constant_pi_6dd0a : Constant  Value=pi
  Product_2a34f : Product
  Product_c6ee4 : Product
  Blockout_d_theta_SG_D_1_9a995 : Outport
  wires:
  State_w_SG_D_1_c5d1e/1 -> Add_b1f62/2
  Constant_-2.0_b7139/1 -> Product_c6ee4/1
  Constant_f0_a2466/1 -> Product_2a34f/2
  Constant_pi_6dd0a/1 -> Product_c6ee4/2
  Product_2a34f/1 -> Add_b1f62/1
  Product_c6ee4/1 -> Product_2a34f/1
  Add_b1f62/1 -> Blockout_d_theta_SG_D_1_9a995/1

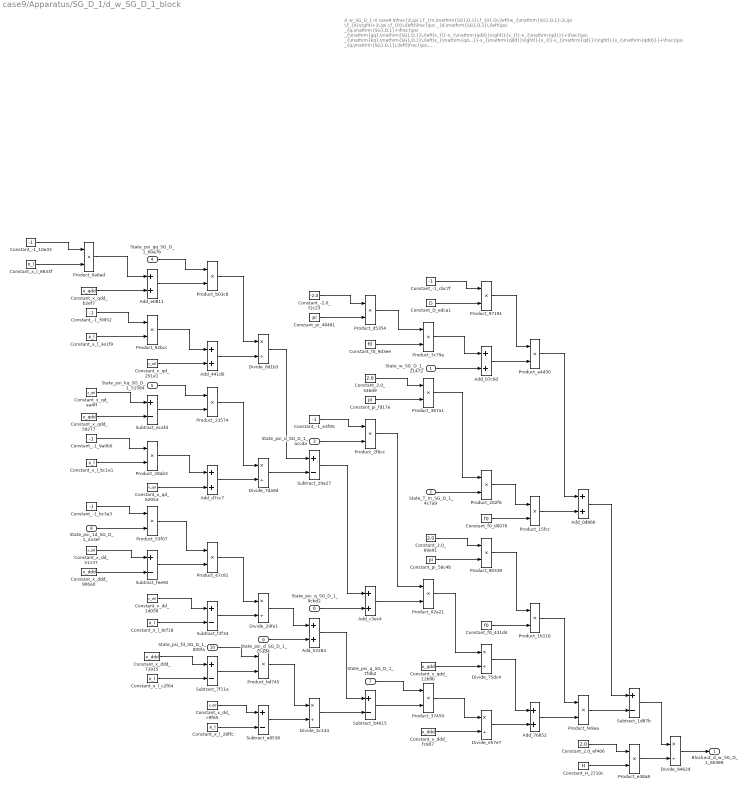
== system case9/Apparatus/SG_D_1/d_w_SG_D_1_block ==
  note: d_w_SG_D_1 in case9
      | $\frac{2\,\pi \,T_{m,\mathrm{SG},D,1}\,f_{0}-D\,\left(w_{\mathrm{SG},D,1}-2\,\pi \,f_{0}\right)+2\,\pi \,f_{0}\,\left(\frac{\psi _{d,\mathrm{SG},D,1}\,\left(\psi _{q,\mathrm{SG},D,1}+\frac{\psi _{\mathrm{gq},\mathrm{SG},D,1}\,\left(x_{l}-x_{\mathrm{qdd}}\right)}{x_{l}-x_{\mathrm{qd}}}+\frac{\psi _{\mathrm{kq},\mathrm{SG},D,1}\,\left(x_{\mathrm{qd}}-x_{\mathrm{qdd}}\right)}{x_{l}-x_{\mathrm{qd}}}\right)}{x_{\mathrm{qdd}}}+\frac{\psi _{q,\mathrm{SG},D,1}\,\left(\frac{\psi _{\mathrm{1d},\mathrm{SG},D,1}\,\left(x_{\mathrm{dd}}-x_{\mathrm{ddd}}\right)}{x_{\mathrm{dd}}-x_{l}}-\psi _{d,\mathrm{SG},D,1}+\frac{\psi _{\mathrm{fd},\mathrm{SG},D,1}\,\left(x_{\mathrm{ddd}}-x_{l}\right)}{x_{\mathrm{dd}}-x_{l}}\right)}{x_{\mathrm{ddd}}}\right)}{2\,H}$
      | Automatically generated on 2025-10-31 19:34:42 .
  State_w_SG_D_1_21472 : Inport
  State_T_m_SG_D_1_4c7a9 : Inport  Port=2
  State_psi_d_SG_D_1_accda : Inport  Port=3
  State_psi_gq_SG_D_1_60a7b : Inport  Port=4
  State_psi_kq_SG_D_1_51584 : Inport  Port=5
  State_psi_q_SG_D_1_9cbd2 : Inport  Port=6
  State_psi_q_SG_D_1_7fdb2 : Inport  Port=7
  State_psi_1d_SG_D_1_2a3ef : Inport  Port=8
  State_psi_d_SG_D_1_c53d4 : Inport  Port=9
  State_psi_fd_SG_D_1_000fa : Inport  Port=10
  Add_07c0d : Sum
  Add_0d866 : Sum
  Add_441d0 : Sum
  Add_52284 : Sum
  Add_76852 : Sum
  Add_c3ec4 : Sum
  Add_d7cc7 : Sum
  Add_e0811 : Sum
  Constant_-1_10e33 : Constant  Value=-1
  Constant_-1_9a0b0 : Constant  Value=-1
  Constant_-1_bc3a3 : Constant  Value=-1
  Constant_-1_cbc7f : Constant  Value=-1
  Constant_-1_e3f05 : Constant  Value=-1
  Constant_-1_f9952 : Constant  Value=-1
  Constant_-2.0_f2c23 : Constant  Value=-2.0
  Constant_2.0_546d9 : Constant  Value=2.0
  Constant_2.0_69e91 : Constant  Value=2.0
  Constant_2.0_ef406 : Constant  Value=2.0
  Constant_D_edca1 : Constant  Value=D
  Constant_H_2710c : Constant  Value=H
  Constant_f0_431d4 : Constant  Value=f0
  Constant_f0_9d3ee : Constant  Value=f0
  Constant_f0_d0076 : Constant  Value=f0
  Constant_pi_48481 : Constant  Value=pi
  Constant_pi_58c4b : Constant  Value=pi
  Constant_pi_fd17e : Constant  Value=pi
  Constant_x_dd_1d058 : Constant  Value=x_dd
  Constant_x_dd_51137 : Constant  Value=x_dd
  Constant_x_dd_c9f65 : Constant  Value=x_dd
  Constant_x_ddd_73915 : Constant  Value=x_ddd
  Constant_x_ddd_906a0 : Constant  Value=x_ddd
  Constant_x_ddd_fc807 : Constant  Value=x_ddd
  Constant_x_l_28ffc : Constant  Value=x_l
  Constant_x_l_3e1f9 : Constant  Value=x_l
  Constant_x_l_8633f : Constant  Value=x_l
  Constant_x_l_8cf18 : Constant  Value=x_l
  Constant_x_l_bc1e1 : Constant  Value=x_l
  Constant_x_l_c2f64 : Constant  Value=x_l
  Constant_x_qd_251e1 : Constant  Value=x_qd
  Constant_x_qd_62054 : Constant  Value=x_qd
  Constant_x_qd_aa4ff : Constant  Value=x_qd
  Constant_x_qdd_12b9b : Constant  Value=x_qdd
  Constant_x_qdd_59277 : Constant  Value=x_qdd
  Constant_x_qdd_b2ef7 : Constant  Value=x_qdd
  Divide_29fe1 : Product  Inputs=*/
  Divide_2c144 : Product  Inputs=*/
  Divide_75dc4 : Product  Inputs=*/
  Divide_7da9d : Product  Inputs=*/
  Divide_8d1b3 : Product  Inputs=*/
  Divide_9462d : Product  Inputs=*/
  Divide_e57e7 : Product  Inputs=*/
  Product_02a21 : Product
  Product_0a6ad : Product
  Product_15fcc : Product
  Product_1b116 : Product
  Product_202f6 : Product
  Product_{23574,37459,90338,97191} (4 alike) : Product
  Product_28ab3 : Product
  Product_2f6cc : Product
  Product_367a1 : Product
  Product_3c79a : Product
  Product_53f07 : Product
  Product_92bcc : Product
  Product_a4d30 : Product
  Product_b03c8 : Product
  Product_bd745 : Product
  Product_d5354 : Product
  Product_e48a8 : Product
  Product_e7c81 : Product
  Product_fe9aa : Product
  Subtract_1d87b : Sum  Inputs=+-
  Subtract_29a27 : Sum  Inputs=+-
  Subtract_7f11a : Sum  Inputs=+-
  Subtract_b4015 : Sum  Inputs=+-
  Subtract_e8538 : Sum  Inputs=+-
  Subtract_ecafd : Sum  Inputs=+-
  Subtract_f2f34 : Sum  Inputs=+-
  Subtract_fee92 : Sum  Inputs=+-
  Blockout_d_w_SG_D_1_60389 : Outport
  wires:
  Product_3c79a/1 -> Add_07c0d/1
  Constant_-1_10e33/1 -> Product_0a6ad/1
  Constant_pi_fd17e/1 -> Product_367a1/2
  Constant_x_qdd_b2ef7/1 -> Add_e0811/2
  Constant_x_l_8633f/1 -> Product_0a6ad/2
  Product_0a6ad/1 -> Add_e0811/1
  Constant_x_qd_aa4ff/1 -> Subtract_ecafd/1
  Constant_-1_f9952/1 -> Product_92bcc/1
  Product_d5354/1 -> Product_3c79a/1
  Constant_x_qdd_59277/1 -> Subtract_ecafd/2
  State_psi_q_SG_D_1_7fdb2/1 -> Product_37459/1
  Constant_x_l_3e1f9/1 -> Product_92bcc/2
  Constant_-1_9a0b0/1 -> Product_28ab3/1
  Constant_x_l_bc1e1/1 -> Product_28ab3/2
  Constant_-1_bc3a3/1 -> Product_53f07/1
  Product_92bcc/1 -> Add_441d0/1
  State_psi_1d_SG_D_1_2a3ef/1 -> Product_53f07/2
  Constant_x_dd_51137/1 -> Subtract_fee92/1
  Subtract_ecafd/1 -> Product_23574/2
  Constant_x_ddd_906a0/1 -> Subtract_fee92/2
  State_psi_gq_SG_D_1_60a7b/1 -> Product_b03c8/1
  Product_2f6cc/1 -> Product_02a21/1
  Add_e0811/1 -> Product_b03c8/2
  Constant_x_qd_251e1/1 -> Add_441d0/2
  State_psi_kq_SG_D_1_51584/1 -> Product_23574/1
  Constant_f0_9d3ee/1 -> Product_3c79a/2
  Product_28ab3/1 -> Add_d7cc7/1
  Constant_x_dd_1d058/1 -> Subtract_f2f34/1
  Constant_x_qd_62054/1 -> Add_d7cc7/2
  Product_53f07/1 -> Product_e7c81/1
  Subtract_fee92/1 -> Product_e7c81/2
  Constant_x_l_8cf18/1 -> Subtract_f2f34/2
  Constant_x_ddd_73915/1 -> Subtract_7f11a/1
  Constant_x_l_c2f64/1 -> Subtract_7f11a/2
  State_w_SG_D_1_21472/1 -> Add_07c0d/2
  Divide_75dc4/1 -> Add_76852/1
  Constant_-1_cbc7f/1 -> Product_97191/1
  Product_b03c8/1 -> Divide_8d1b3/1
  Add_07c0d/1 -> Product_a4d30/2
  Divide_8d1b3/1 -> Subtract_29a27/1
  Add_441d0/1 -> Divide_8d1b3/2
  Constant_pi_48481/1 -> Product_d5354/2
  Product_23574/1 -> Divide_7da9d/1
  Add_d7cc7/1 -> Divide_7da9d/2
  Product_e7c81/1 -> Divide_29fe1/1
  Divide_29fe1/1 -> Add_52284/1
  Subtract_f2f34/1 -> Divide_29fe1/2
  State_psi_fd_SG_D_1_000fa/1 -> Product_bd745/1
  Subtract_7f11a/1 -> Product_bd745/2
  Constant_x_dd_c9f65/1 -> Subtract_e8538/1
  Constant_x_l_28ffc/1 -> Subtract_e8538/2
  Divide_7da9d/1 -> Subtract_29a27/2
  Constant_2.0_546d9/1 -> Product_367a1/1
  State_psi_d_SG_D_1_c53d4/1 -> Add_52284/2
  Product_bd745/1 -> Divide_2c144/1
  Subtract_e8538/1 -> Divide_2c144/2
  Constant_-2.0_f2c23/1 -> Product_d5354/1
  Constant_-1_e3f05/1 -> Product_2f6cc/1
  State_psi_d_SG_D_1_accda/1 -> Product_2f6cc/2
  Subtract_29a27/1 -> Add_c3ec4/1
  Subtract_b4015/1 -> Product_37459/2
  State_psi_q_SG_D_1_9cbd2/1 -> Add_c3ec4/2
  Add_52284/1 -> Subtract_b4015/1
  Divide_2c144/1 -> Subtract_b4015/2
  Add_c3ec4/1 -> Product_02a21/2
  Constant_D_edca1/1 -> Product_97191/2
  Product_367a1/1 -> Product_202f6/1
  State_T_m_SG_D_1_4c7a9/1 -> Product_202f6/2
  Constant_2.0_69e91/1 -> Product_90338/1
  Constant_pi_58c4b/1 -> Product_90338/2
  Product_02a21/1 -> Divide_75dc4/1
  Constant_x_qdd_12b9b/1 -> Divide_75dc4/2
  Product_37459/1 -> Divide_e57e7/1
  Constant_x_ddd_fc807/1 -> Divide_e57e7/2
  Product_97191/1 -> Product_a4d30/1
  Product_202f6/1 -> Product_15fcc/1
  Constant_f0_d0076/1 -> Product_15fcc/2
  Product_90338/1 -> Product_1b116/1
  Constant_f0_431d4/1 -> Product_1b116/2
  Divide_e57e7/1 -> Add_76852/2
  Product_a4d30/1 -> Add_0d866/1
  Product_15fcc/1 -> Add_0d866/2
  Product_1b116/1 -> Product_fe9aa/1
  Add_76852/1 -> Product_fe9aa/2
  Add_0d866/1 -> Subtract_1d87b/1
  Product_fe9aa/1 -> Subtract_1d87b/2
  Constant_2.0_ef406/1 -> Product_e48a8/1
  Constant_H_2710c/1 -> Product_e48a8/2
  Subtract_1d87b/1 -> Divide_9462d/1
  Product_e48a8/1 -> Divide_9462d/2
  Divide_9462d/1 -> Blockout_d_w_SG_D_1_60389/1

== system case9/Apparatus/SG_D_1/i_d_SG_D_1_block ==
  note: i_d_SG_D_1 in case9
      | $\frac{\sin\left(\theta _{\mathrm{SG},D,1}\right)\,\left(\frac{\psi _{\mathrm{1d},\mathrm{SG},D,1}\,\left(x_{\mathrm{dd}}-x_{\mathrm{ddd}}\right)}{x_{\mathrm{dd}}-x_{l}}-\psi _{d,\mathrm{SG},D,1}+\frac{\psi _{\mathrm{fd},\mathrm{SG},D,1}\,\left(x_{\mathrm{ddd}}-x_{l}\right)}{x_{\mathrm{dd}}-x_{l}}\right)}{x_{\mathrm{ddd}}}-\frac{\cos\left(\theta _{\mathrm{SG},D,1}\right)\,\left(\psi _{q,\mathrm{SG},D,1}+\frac{\psi _{\mathrm{gq},\mathrm{SG},D,1}\,\left(x_{l}-x_{\mathrm{qdd}}\right)}{x_{l}-x_{\mathrm{qd}}}+\frac{\psi _{\mathrm{kq},\mathrm{SG},D,1}\,\left(x_{\mathrm{qd}}-x_{\mathrm{qdd}}\right)}{x_{l}-x_{\mathrm{qd}}}\right)}{x_{\mathrm{qdd}}}$
      | Automatically generated on 2025-10-31 19:34:48 .
  State_psi_gq_SG_D_1_5e903 : Inport
  State_psi_kq_SG_D_1_6f9a9 : Inport  Port=2
  State_psi_q_SG_D_1_9d632 : Inport  Port=3
  State_theta_SG_D_1_64896 : Inport  Port=4
  State_psi_1d_SG_D_1_fc20b : Inport  Port=5
  State_psi_d_SG_D_1_e0cb1 : Inport  Port=6
  State_psi_fd_SG_D_1_adb2f : Inport  Port=7
  State_theta_SG_D_1_13345 : Inport  Port=8
  Add_247ea : Sum
  Add_286a6 : Sum
  Add_31990 : Sum
  Add_454cc : Sum
  Add_4a189 : Sum
  Constant_-1_076d5 : Constant  Value=-1
  Constant_-1_4d312 : Constant  Value=-1
  Constant_-1_4d5c4 : Constant  Value=-1
  Constant_-1_5976c : Constant  Value=-1
  Constant_-1_dd124 : Constant  Value=-1
  Constant_x_dd_007e6 : Constant  Value=x_dd
  Constant_x_dd_c34a3 : Constant  Value=x_dd
  Constant_x_dd_f0881 : Constant  Value=x_dd
  Constant_x_ddd_110d2 : Constant  Value=x_ddd
  Constant_x_ddd_72aea : Constant  Value=x_ddd
  Constant_x_ddd_be748 : Constant  Value=x_ddd
  Constant_x_l_2cf29 : Constant  Value=x_l
  Constant_x_l_33cfc : Constant  Value=x_l
  Constant_x_l_80225 : Constant  Value=x_l
  Constant_x_l_87e71 : Constant  Value=x_l
  Constant_x_l_90c1c : Constant  Value=x_l
  Constant_x_l_cf6c4 : Constant  Value=x_l
  Constant_x_qd_a7920 : Constant  Value=x_qd
  Constant_x_qd_aca68 : Constant  Value=x_qd
  Constant_x_qd_f226c : Constant  Value=x_qd
  Constant_x_qdd_20bca : Constant  Value=x_qdd
  Constant_x_qdd_461a0 : Constant  Value=x_qdd
  Constant_x_qdd_877bd : Constant  Value=x_qdd
  Divide_5b3c5 : Product  Inputs=*/
  Divide_5be62 : Product  Inputs=*/
  Divide_a6967 : Product  Inputs=*/
  Divide_c3a12 : Product  Inputs=*/
  Divide_e972b : Product  Inputs=*/
  Divide_ec40b : Product  Inputs=*/
  MathFunc_cos_b3de4 : Trigonometry  Operator=cos
  MathFunc_sin_2e09c : Trigonometry
  Product_08764 : Product
  Product_2a53a : Product
  Product_30789 : Product
  Product_581db : Product
  Product_7c7f7 : Product
  Product_86e8f : Product
  Product_961ec : Product
  Product_b086f : Product
  Product_c95e9 : Product
  Product_e0b4f : Product
  Product_fddf1 : Product
  Subtract_00ba0 : Sum  Inputs=+-
  Subtract_08930 : Sum  Inputs=+-
  Subtract_302f4 : Sum  Inputs=+-
  Subtract_665bc : Sum  Inputs=+-
  Subtract_6b100 : Sum  Inputs=+-
  Subtract_8c077 : Sum  Inputs=+-
  Subtract_9df1f : Sum  Inputs=+-
  Subtract_d9b99 : Sum  Inputs=+-
  Blockout_i_d_SG_D_1_272fd : Outport
  wires:
  Constant_-1_4d5c4/1 -> Product_fddf1/1
  Constant_x_l_90c1c/1 -> Product_fddf1/2
  Constant_x_ddd_be748/1 -> Subtract_665bc/2
  Product_fddf1/1 -> Add_454cc/1
  Constant_x_qdd_20bca/1 -> Subtract_08930/2
  Constant_x_l_33cfc/1 -> Product_e0b4f/2
  Constant_x_qd_a7920/1 -> Add_247ea/2
  Constant_x_qdd_877bd/1 -> Add_454cc/2
  Constant_x_qd_aca68/1 -> Subtract_08930/1
  MathFunc_cos_b3de4/1 -> Product_581db/2
  Constant_-1_076d5/1 -> Product_e0b4f/1
  Constant_-1_dd124/1 -> Product_30789/1
  Subtract_d9b99/1 -> Blockout_i_d_SG_D_1_272fd/1
  Constant_x_l_80225/1 -> Product_30789/2
  Divide_a6967/1 -> Subtract_8c077/1
  State_psi_gq_SG_D_1_5e903/1 -> Product_2a53a/1
  Subtract_302f4/1 -> Product_7c7f7/2
  Add_454cc/1 -> Product_2a53a/2
  Divide_5b3c5/1 -> Add_4a189/1
  Product_e0b4f/1 -> Add_31990/1
  Constant_x_qd_f226c/1 -> Add_31990/2
  State_psi_kq_SG_D_1_6f9a9/1 -> Product_b086f/1
  Add_4a189/1 -> Subtract_00ba0/1
  Add_31990/1 -> Divide_a6967/2
  Subtract_08930/1 -> Product_b086f/2
  Product_30789/1 -> Add_247ea/1
  Constant_-1_4d312/1 -> Product_86e8f/1
  State_psi_1d_SG_D_1_fc20b/1 -> Product_86e8f/2
  Constant_x_dd_f0881/1 -> Subtract_665bc/1
  Product_2a53a/1 -> Divide_a6967/1
  Product_08764/1 -> Divide_c3a12/1
  Subtract_665bc/1 -> Product_c95e9/2
  Product_b086f/1 -> Divide_e972b/1
  Product_86e8f/1 -> Product_c95e9/1
  Add_247ea/1 -> Divide_e972b/2
  Constant_x_dd_007e6/1 -> Subtract_6b100/1
  Subtract_8c077/1 -> Add_286a6/1
  Constant_x_l_cf6c4/1 -> Subtract_6b100/2
  Constant_x_ddd_110d2/1 -> Subtract_302f4/1
  Constant_x_l_2cf29/1 -> Subtract_302f4/2
  Divide_c3a12/1 -> Subtract_d9b99/2
  Divide_e972b/1 -> Subtract_8c077/2
  State_theta_SG_D_1_64896/1 -> MathFunc_cos_b3de4/1
  Product_c95e9/1 -> Divide_5b3c5/1
  Subtract_6b100/1 -> Divide_5b3c5/2
  State_theta_SG_D_1_13345/1 -> MathFunc_sin_2e09c/1
  State_psi_fd_SG_D_1_adb2f/1 -> Product_7c7f7/1
  Constant_x_dd_c34a3/1 -> Subtract_9df1f/1
  Constant_x_l_87e71/1 -> Subtract_9df1f/2
  State_psi_q_SG_D_1_9d632/1 -> Add_286a6/2
  State_psi_d_SG_D_1_e0cb1/1 -> Add_4a189/2
  Constant_x_ddd_72aea/1 -> Divide_c3a12/2
  MathFunc_sin_2e09c/1 -> Product_08764/2
  Product_7c7f7/1 -> Divide_5be62/1
  Constant_-1_5976c/1 -> Product_961ec/1
  Subtract_9df1f/1 -> Divide_5be62/2
  Add_286a6/1 -> Product_961ec/2
  Divide_5be62/1 -> Subtract_00ba0/2
  Product_961ec/1 -> Product_581db/1
  Subtract_00ba0/1 -> Product_08764/1
  Constant_x_qdd_461a0/1 -> Divide_ec40b/2
  Product_581db/1 -> Divide_ec40b/1
  Divide_ec40b/1 -> Subtract_d9b99/1
